simulink model "reaction_wheel"  (R2023b)
settings: Solver=ode4  StartTime=t0  StopTime=tf  FixedStep=t_step  RelTol=1e-3
values from neighbouring files (symbols this model uses):
  A = eye(3)    [reaction_wheels_code.m]
  A_inv = inv(A)    [reaction_wheels_code.m]
  h_r_0 = [0 0 0]'    [reaction_wheels_code.m]
  I = [Ix 0 0; 0 Iy 0; 0 0 Iz]    [orbita.m]    (also in reaction_wheels_code.m)
  I_inv = inv(I)    [orbita.m]    (also in reaction_wheels_code.m)
  I_RW = 1*10^(-5)    (= 1e-05)    [reaction_wheels_code.m]
  I_vector_RW = [I_RW I_RW I_RW]'    [reaction_wheels_code.m]
  M = 0    [orbita.m]    (also in reaction_wheels_code.m)
  omega_0 = [0.45 0.52 0.55]'    [orbita.m]    (also in reaction_wheels_code.m = [0 0 0]')
  t_step = 0.1    [reaction_wheels_code.m]
  w0_RW = [0 0 0]    [reaction_wheels_code.m]
  wMax_RW = 2*pi * RPM_max_RW / 60    (= 527.263967027)    [reaction_wheels_code.m]
libraries: simulink x3, matrix_library x2
settings Model: Creator=valen  LastModifiedBy=samue

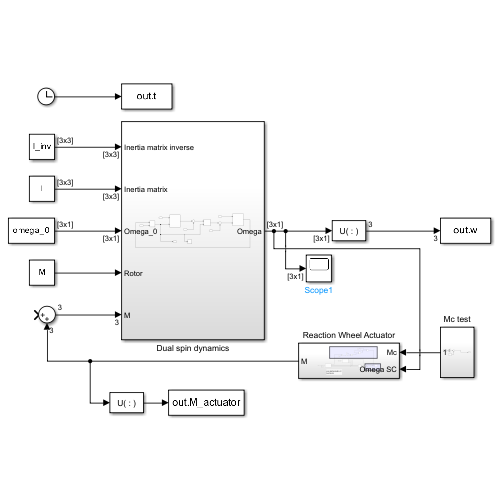
[thumbnail: Simulink's stored preview of the top-level diagram]
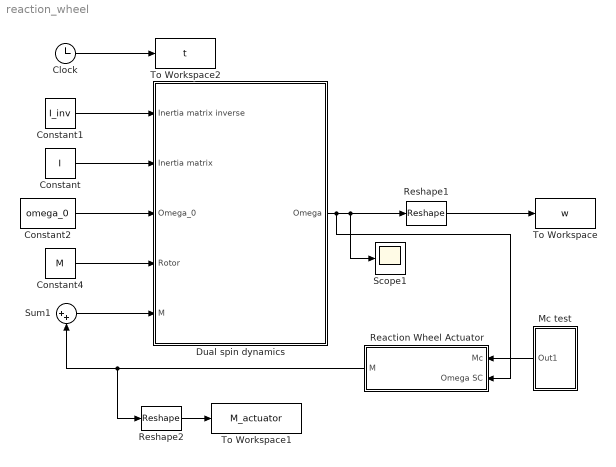
== system reaction_wheel ==
  Clock : Clock
  Constant : Constant  Value=I  VectorParams1D=off
  Constant1 : Constant  Value=I_inv  VectorParams1D=off
  Constant2 : Constant  Value=omega_0  VectorParams1D=off
  Constant4 : Constant  Value=M  VectorParams1D=off
  Dual spin dynamics : Subsystem
  Mc test : Subsystem
  Reaction Wheel Actuator : Subsystem
  Reshape1 : Reshape
  Reshape2 : Reshape
  Scope1 : Scope
  Sum1 : Sum  Inputs=|++
  To Workspace : ToWorkspace  VariableName=w  SampleTime=-1
  To Workspace1 : ToWorkspace  VariableName=M_actuator  SampleTime=-1
  To Workspace2 : ToWorkspace  VariableName=t  SampleTime=-1
  wires:
  Constant/1 -> Dual spin dynamics/2(Inertia matrix)
  Constant2/1 -> Dual spin dynamics/3(Omega_0)
  Clock/1 -> To Workspace2/1
  Reaction Wheel Actuator/1(M) -> Reshape2/1, Sum1/2
  Constant4/1 -> Dual spin dynamics/4(Rotor)
  Sum1/1 -> Dual spin dynamics/5(M)
  Constant1/1 -> Dual spin dynamics/1(Inertia matrix inverse)
  Dual spin dynamics/1(Omega) -> Reshape1/1, Scope1/1, Reaction Wheel Actuator/2(Omega SC)
  Reshape1/1 -> To Workspace/1
  Mc test/1(Out1) -> Reaction Wheel Actuator/1(Mc)
  Reshape2/1 -> To Workspace1/1

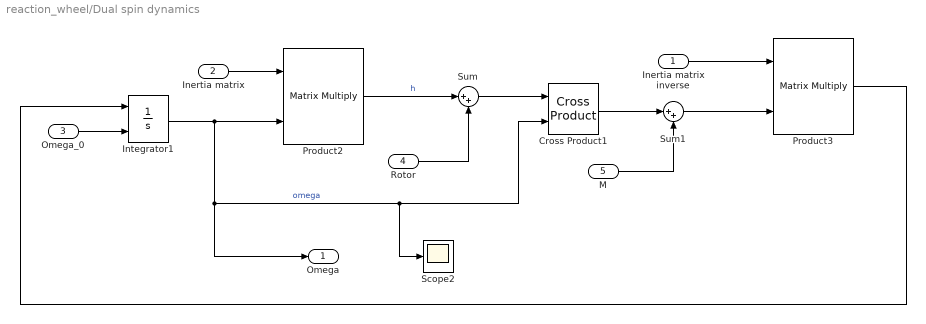
== system reaction_wheel/Dual spin dynamics ==
  Inertia matrix inverse : Inport
  Inertia matrix : Inport  Port=2
  Omega_0 : Inport  Port=3
  Rotor : Inport  Port=4
  M : Inport  Port=5
  Cross Product1 : matrix_library/Cross Product
  Integrator1 : Integrator  InitialConditionSource=external
  Product2 : Product  Multiplication=Matrix(*)
  Product3 : Product  Multiplication=Matrix(*)
  Scope2 : Scope
  Sum : Sum  Inputs=|++
  Sum1 : Sum  Inputs=|++
  Omega : Outport
  wires:
  M/1 -> Sum1/2
  Sum1/1 -> Product3/2
  Omega_0/1 -> Integrator1/2
  Product2/1 -> Sum/1  "h"
  Inertia matrix/1 -> Product2/1
  Product3/1 -> Integrator1/1
  Rotor/1 -> Sum/2
  Integrator1/1 -> Product2/2, Omega/1, Scope2/1, Cross Product1/2  "omega"
  Cross Product1/1 -> Sum1/1
  Inertia matrix inverse/1 -> Product3/1
  Sum/1 -> Cross Product1/1

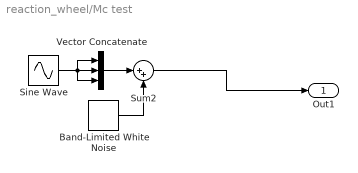
== system reaction_wheel/Mc test ==
  Band-Limited White Noise : simulink/Sources/Band-Limited White Noise  Cov=[0.00001]  Ts=t_step  seed=[23341]
  Sine Wave : Sin  Amplitude=0.003  Frequency=0.1  SampleTime=2
  Sum2 : Sum  Inputs=|++
  Vector Concatenate : Concatenate  NumInputs=3
  Out1 : Outport
  wires:
  Band-Limited White Noise/1 -> Sum2/2
  Sine Wave/1 -> Vector Concatenate/2, Vector Concatenate/1, Vector Concatenate/3
  Vector Concatenate/1 -> Sum2/1
  Sum2/1 -> Out1/1

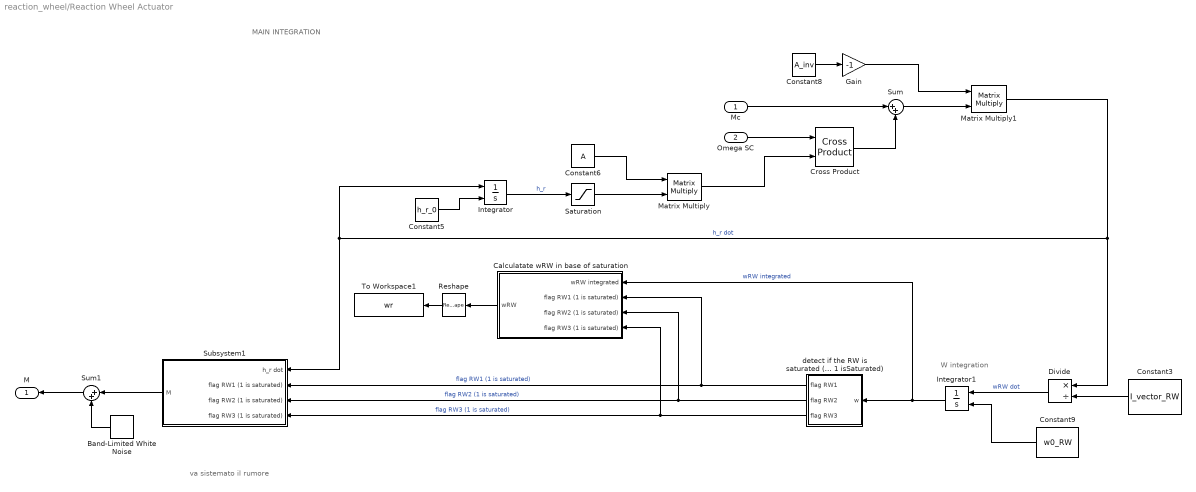
== system reaction_wheel/Reaction Wheel Actuator ==
  note: W integration
  note: va sistemato il rumore
  note: MAIN INTEGRATION
  Mc : Inport
  Omega SC : Inport  Port=2
  Band-Limited White Noise : simulink/Sources/Band-Limited White Noise  Cov=[0.00001]  Ts=t_step  seed=[23341]
  Calculatate wRW in base of saturation : Subsystem
  Constant3 : Constant  Value=I_vector_RW
  Constant5 : Constant  Value=h_r_0  VectorParams1D=off
  Constant6 : Constant  Value=A  VectorParams1D=off
  Constant8 : Constant  Value=A_inv  VectorParams1D=off
  Constant9 : Constant  Value=w0_RW
  Cross Product : matrix_library/Cross Product
  Divide : Product  Inputs=*/
  Gain : Gain  Gain=-1
  Integrator : Integrator  InitialConditionSource=external
  Integrator1 : Integrator  InitialConditionSource=external
  Matrix Multiply : Product  Multiplication=Matrix(*)
  Matrix Multiply1 : Product  Multiplication=Matrix(*)
  Reshape : Reshape
  Saturation : Saturate  UpperLimit=wMax_RW*I_RW  LowerLimit=-wMax_RW*I_RW
  Subsystem1 : Subsystem
  Sum : Sum  Inputs=|++
  Sum1 : Sum  Inputs=|++
  To Workspace1 : ToWorkspace  VariableName=wr  SampleTime=-1
  detect if the RW is saturated (output == 1 isSaturated) : Subsystem
  M : Outport
  wires:
  Matrix Multiply1/1 -> Integrator/1, Subsystem1/1(h_r dot), Divide/1  "h_r dot"
  Constant6/1 -> Matrix Multiply/1
  Cross Product/1 -> Sum/2
  Constant8/1 -> Gain/1
  Sum/1 -> Matrix Multiply1/2
  detect if the RW is saturated (output == 1 isSaturated)/2(flag RW2) -> Calculatate wRW in base of saturation/3(flag RW2 (1 is saturated)), Subsystem1/3(flag RW2 (1 is saturated))  "flag RW2 (1 is saturated)"
  Calculatate wRW in base of saturation/1(wRW) -> Reshape/1
  Matrix Multiply/1 -> Cross Product/2
  Constant5/1 -> Integrator/2
  Constant3/1 -> Divide/2
  Gain/1 -> Matrix Multiply1/1
  Mc/1 -> Sum/1
  Saturation/1 -> Matrix Multiply/2
  Integrator1/1 -> Calculatate wRW in base of saturation/1(wRW integrated), detect if the RW is saturated (output == 1 isSaturated)/1(w)  "wRW integrated"
  Constant9/1 -> Integrator1/2
  Divide/1 -> Integrator1/1  "wRW dot"
  Integrator/1 -> Saturation/1  "h_r"
  detect if the RW is saturated (output == 1 isSaturated)/3(flag RW3) -> Calculatate wRW in base of saturation/4(flag RW3 (1 is saturated)), Subsystem1/4(flag RW3 (1 is saturated))  "flag RW3 (1 is saturated)"
  detect if the RW is saturated (output == 1 isSaturated)/1(flag RW1) -> Calculatate wRW in base of saturation/2(flag RW1 (1 is saturated)), Subsystem1/2(flag RW1 (1 is saturated))  "flag RW1 (1 is saturated)"
  Reshape/1 -> To Workspace1/1
  Omega SC/1 -> Cross Product/1
  Subsystem1/1(M) -> Sum1/1
  Sum1/1 -> M/1
  Band-Limited White Noise/1 -> Sum1/2

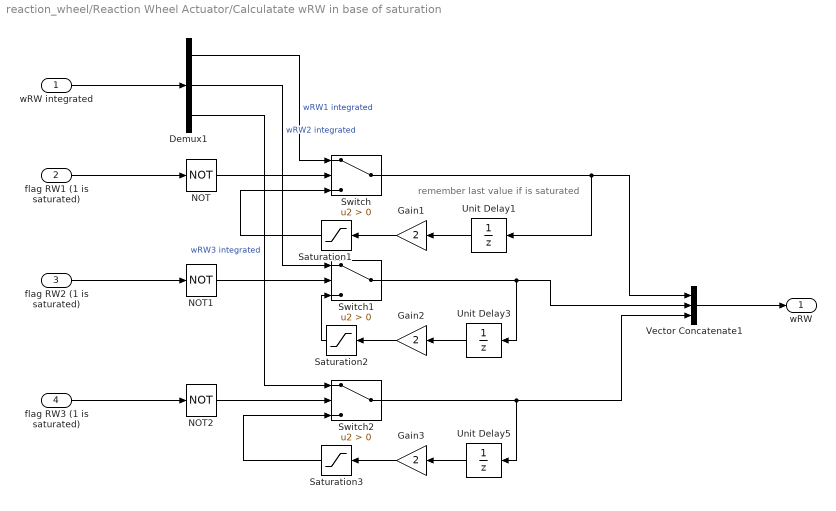
== system reaction_wheel/Reaction Wheel Actuator/Calculatate wRW in base of saturation ==
  note: remember last value if is saturated
  wRW integrated : Inport
  flag RW1 (1 is saturated) : Inport  Port=2
  flag RW2 (1 is saturated) : Inport  Port=3
  flag RW3 (1 is saturated) : Inport  Port=4
  Demux1 : Demux  Outputs=3
  Gain1 : Gain  Gain=2
  Gain2 : Gain  Gain=2
  Gain3 : Gain  Gain=2
  NOT : Logic  Operator=NOT  IconShape=distinctive  AllPortsSameDT=off  OutDataTypeStr=boolean
  NOT1 : Logic  Operator=NOT  IconShape=distinctive  AllPortsSameDT=off  OutDataTypeStr=boolean
  NOT2 : Logic  Operator=NOT  IconShape=distinctive  AllPortsSameDT=off  OutDataTypeStr=boolean
  Saturation1 : Saturate  UpperLimit=wMax_RW  LowerLimit=-wMax_RW
  Saturation2 : Saturate  UpperLimit=wMax_RW  LowerLimit=-wMax_RW
  Saturation3 : Saturate  UpperLimit=wMax_RW  LowerLimit=-wMax_RW
  Switch : Switch  Criteria=u2 > Threshold  SaturateOnIntegerOverflow=off  InputSameDT=off
  Switch1 : Switch  Criteria=u2 > Threshold  SaturateOnIntegerOverflow=off  InputSameDT=off
  Switch2 : Switch  Criteria=u2 > Threshold  SaturateOnIntegerOverflow=off  InputSameDT=off
  Unit Delay1 : UnitDelay  SampleTime=-1  HasFrameUpgradeWarning=on
  Unit Delay3 : UnitDelay  SampleTime=-1  HasFrameUpgradeWarning=on
  Unit Delay5 : UnitDelay  SampleTime=-1  HasFrameUpgradeWarning=on
  Vector Concatenate1 : Concatenate  NumInputs=3
  wRW : Outport
  wires:
  Gain2/1 -> Saturation2/1
  Switch1/1 -> Unit Delay3/1, Vector Concatenate1/2
  NOT/1 -> Switch/2
  flag RW1 (1 is saturated)/1 -> NOT/1
  Saturation3/1 -> Switch2/3
  NOT1/1 -> Switch1/2
  Saturation2/1 -> Switch1/3
  wRW integrated/1 -> Demux1/1
  Switch2/1 -> Unit Delay5/1, Vector Concatenate1/3
  Unit Delay5/1 -> Gain3/1
  Unit Delay3/1 -> Gain2/1
  Demux1/2 -> Switch1/1  "wRW2 integrated"
  Gain1/1 -> Saturation1/1
  Vector Concatenate1/1 -> wRW/1
  Switch/1 -> Unit Delay1/1, Vector Concatenate1/1
  Unit Delay1/1 -> Gain1/1
  Saturation1/1 -> Switch/3
  Demux1/3 -> Switch2/1  "wRW3 integrated"
  Demux1/1 -> Switch/1  "wRW1 integrated"
  NOT2/1 -> Switch2/2
  Gain3/1 -> Saturation3/1
  flag RW3 (1 is saturated)/1 -> NOT2/1
  flag RW2 (1 is saturated)/1 -> NOT1/1

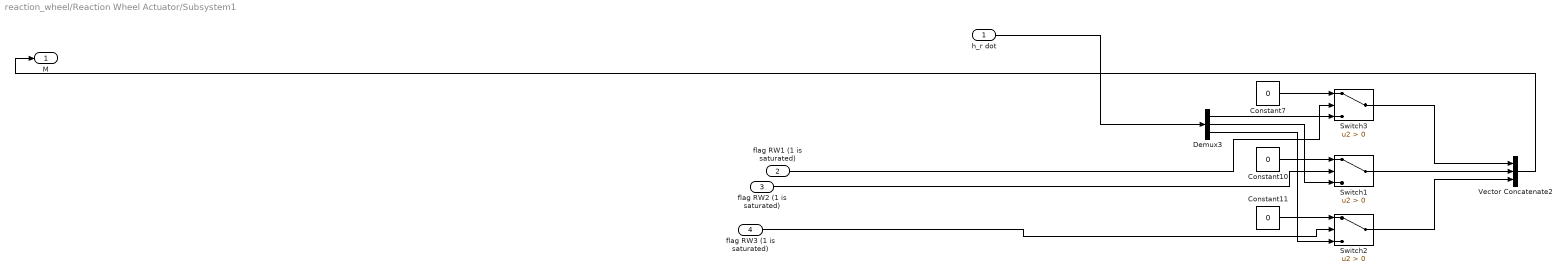
== system reaction_wheel/Reaction Wheel Actuator/Subsystem1 ==
  h_r dot : Inport
  flag RW1 (1 is saturated) : Inport  Port=2
  flag RW2 (1 is saturated) : Inport  Port=3
  flag RW3 (1 is saturated) : Inport  Port=4
  Constant10 : Constant  Value=0
  Constant11 : Constant  Value=0
  Constant7 : Constant  Value=0
  Demux3 : Demux  Outputs=3
  Switch1 : Switch  Criteria=u2 > Threshold  SaturateOnIntegerOverflow=off  InputSameDT=off
  Switch2 : Switch  Criteria=u2 > Threshold  SaturateOnIntegerOverflow=off  InputSameDT=off
  Switch3 : Switch  Criteria=u2 > Threshold  SaturateOnIntegerOverflow=off  InputSameDT=off
  Vector Concatenate2 : Concatenate  NumInputs=3
  M : Outport
  wires:
  Demux3/3 -> Switch2/3
  Constant11/1 -> Switch2/1
  Switch2/1 -> Vector Concatenate2/3
  Demux3/1 -> Switch3/3
  Demux3/2 -> Switch1/3
  Switch3/1 -> Vector Concatenate2/1
  Switch1/1 -> Vector Concatenate2/2
  flag RW3 (1 is saturated)/1 -> Switch2/2
  Constant7/1 -> Switch3/1
  Constant10/1 -> Switch1/1
  flag RW1 (1 is saturated)/1 -> Switch3/2
  h_r dot/1 -> Demux3/1
  flag RW2 (1 is saturated)/1 -> Switch1/2
  Vector Concatenate2/1 -> M/1

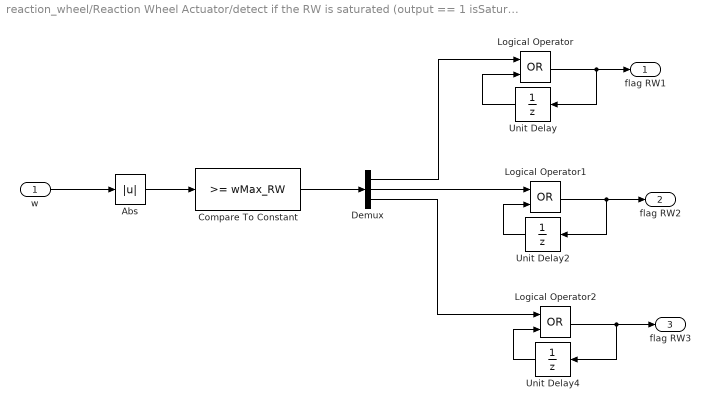
== system reaction_wheel/Reaction Wheel Actuator/detect if the RW is saturated (output == 1 isSaturated) ==
  w : Inport
  Abs : Abs  SaturateOnIntegerOverflow=off
  Compare To Constant : simulink/Logic and Bit Operations/Compare To Constant  relop=>=  const=wMax_RW  OutDataTypeStr=boolean
  Demux : Demux  Outputs=3
  Logical Operator : Logic  Operator=OR  AllPortsSameDT=off  OutDataTypeStr=boolean
  Logical Operator1 : Logic  Operator=OR  AllPortsSameDT=off  OutDataTypeStr=boolean
  Logical Operator2 : Logic  Operator=OR  AllPortsSameDT=off  OutDataTypeStr=boolean
  Unit Delay : UnitDelay  SampleTime=-1  HasFrameUpgradeWarning=on
  Unit Delay2 : UnitDelay  SampleTime=-1  HasFrameUpgradeWarning=on
  Unit Delay4 : UnitDelay  SampleTime=-1  HasFrameUpgradeWarning=on
  flag RW1 : Outport
  flag RW2 : Outport  Port=2
  flag RW3 : Outport  Port=3
  wires:
  Unit Delay4/1 -> Logical Operator2/2
  Unit Delay/1 -> Logical Operator/2
  Demux/1 -> Logical Operator/1
  Logical Operator/1 -> flag RW1/1, Unit Delay/1
  Unit Delay2/1 -> Logical Operator1/2
  Logical Operator2/1 -> flag RW3/1, Unit Delay4/1
  Demux/2 -> Logical Operator1/1
  Logical Operator1/1 -> flag RW2/1, Unit Delay2/1
  Demux/3 -> Logical Operator2/1
  Abs/1 -> Compare To Constant/1
  w/1 -> Abs/1
  Compare To Constant/1 -> Demux/1
